simulink model "fomodel_w_P_control"  (R2019b)
settings: Solver=VariableStepAuto  StartTime=0.0  StopTime=8  RelTol=1e-3
values from neighbouring files (symbols this model uses):
  K_p = 0.5    [Question_3_2.m]    (also in Question_3_3.m = 1)
  K_v = 96    [K_v_and_tau_v.mat]    (also in Question_3_1.m; Question_3_3.m)
  tau_v = 0.0965    [K_v_and_tau_v.mat]    (also in Question_3_1.m; Question_3_3.m)
settings Model: Creator=johns  LastModifiedBy=johns

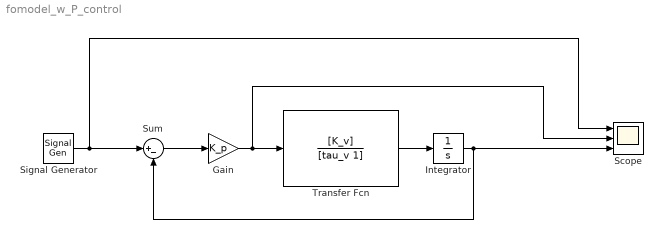
== system fomodel_w_P_control ==
  Gain : Gain  Gain=K_p
  Integrator : Integrator
  Scope : Scope  NumInputPorts=3
  Signal Generator : SignalGenerator  Amplitude=5  Frequency=0.5
  Sum : Sum  Inputs=|+-
  Transfer Fcn : TransferFcn  Numerator=[K_v]  Denominator=[tau_v 1]
  wires:
  Signal Generator/1 -> Scope/1, Sum/1
  Sum/1 -> Gain/1
  Transfer Fcn/1 -> Integrator/1
  Gain/1 -> Scope/2, Transfer Fcn/1
  Integrator/1 -> Scope/3, Sum/2
